simulink model "CM640C_MotAg1Meas"  (R2013b)
settings: Solver=VariableStepDiscrete  SolverMode=SingleTasking  StartTime=0.0  StopTime=1  FixedStep=0.002  RelTol=1e-3
values from neighbouring files (symbols this model uses):
  ARCHGLBPRM_2PI_ULS_F32 = DataDict.Constant    [CM640C_MotAg1Meas_DataDict.m]
  CNTPERREV_MOTREV_S15P16 = DataDict.Constant    [CM640C_MotAg1Meas_DataDict.m]
  COEFFTBLELMSIZE_CNT_U08 = DataDict.Constant    [CM640C_MotAg1Meas_DataDict.m]
  COEFFTBLSIZE_CNT_U08 = DataDict.Constant    [CM640C_MotAg1Meas_DataDict.m]
  CORRNTBLAGSTEPSIZE_MATRAD_F32 = DataDict.Constant    [CM640C_MotAg1Meas_DataDict.m]
  CORRNTBLSIDXOFFS_CNT_U16 = DataDict.Constant    [CM640C_MotAg1Meas_DataDict.m]
  CORRNTBLSIZE_CNT_U16 = DataDict.Constant    [CM640C_MotAg1Meas_DataDict.m]
  CORRNTBLSIZEMASK_CNT_U08 = DataDict.Constant    [CM640C_MotAg1Meas_DataDict.m]
  MOTAG1ERRTHD_MOTREV_U0P16 = DataDict.Constant    [CM640C_MotAg1Meas_DataDict.m]
  MotAg1MeasMotAgOffs = DataDict.Calibration    [CM640C_MotAg1Meas_DataDict.m]
  MotAg1PrtclFlt = DataDict.NTC    [CM640C_MotAg1Meas_DataDict.m]
  MOTAG1PRTCLFLTFAILSTEP_CNT_U16 = DataDict.Constant    [CM640C_MotAg1Meas_DataDict.m]
  MOTAG1PRTCLFLTPASSSTEP_CNT_U16 = DataDict.Constant    [CM640C_MotAg1Meas_DataDict.m]
  MOTAGCPTLIMFLTMASK_CNT_U32 = DataDict.Constant    [CM640C_MotAg1Meas_DataDict.m]
  MOTAGDELTAPERCORRNPT_CNT_U16 = DataDict.Constant    [CM640C_MotAg1Meas_DataDict.m]
  MOTAGFLTMASK_CNT_U32 = DataDict.Constant    [CM640C_MotAg1Meas_DataDict.m]
  MOTAGIDXMASK_CNT_U16 = DataDict.Constant    [CM640C_MotAg1Meas_DataDict.m]
  MOTAGLIMMASK_CNT_S32 = DataDict.Constant    [CM640C_MotAg1Meas_DataDict.m]
  MOTAGMGNLIMFLTMASK_CNT_U32 = DataDict.Constant    [CM640C_MotAg1Meas_DataDict.m]
  MOTAGMINWAITPERD_CNT_U32 = DataDict.Constant    [CM640C_MotAg1Meas_DataDict.m]
  MOTAGOFFS_CNT_S32 = DataDict.Constant    [CM640C_MotAg1Meas_DataDict.m]
  MOTAGOVFFLTMASK_CNT_U32 = DataDict.Constant    [CM640C_MotAg1Meas_DataDict.m]
  MOTAGSPITRSMMASK_CNT_U32 = DataDict.Constant    [CM640C_MotAg1Meas_DataDict.m]
  MOTAGVLTGFLTMASK_CNT_U32 = DataDict.Constant    [CM640C_MotAg1Meas_DataDict.m]
  NOMOTAGFLTMASK_CNT_U32 = DataDict.Constant    [CM640C_MotAg1Meas_DataDict.m]
  READBUFADR_CNT_U32 = DataDict.Constant    [CM640C_MotAg1Meas_DataDict.m]
  READBUFIDX_CNT_U08 = DataDict.Constant    [CM640C_MotAg1Meas_DataDict.m]
  SNSRAGMASK_CNT_U32 = DataDict.Constant    [CM640C_MotAg1Meas_DataDict.m]
  SNSRCNTMASK_CNT_U32 = DataDict.Constant    [CM640C_MotAg1Meas_DataDict.m]
  SPIAGCNTREGIDX_CNT_U08 = DataDict.Constant    [CM640C_MotAg1Meas_DataDict.m]
  SPIAGREGIDX_CNT_U08 = DataDict.Constant    [CM640C_MotAg1Meas_DataDict.m]
  SPISTATREGIDX_CNT_U08 = DataDict.Constant    [CM640C_MotAg1Meas_DataDict.m]
  SPITURNCNTRREGIDX_CNT_U08 = DataDict.Constant    [CM640C_MotAg1Meas_DataDict.m]
  STRTPTRINITVAL_CNT_U32 = DataDict.Constant    [CM640C_MotAg1Meas_DataDict.m]
  STRTPTRPERVAL_CNT_U32 = DataDict.Constant    [CM640C_MotAg1Meas_DataDict.m]
  TURNCNTRHALFOFFS_CNT_S16 = DataDict.Constant    [CM640C_MotAg1Meas_DataDict.m]
  TURNCNTROFFS_CNT_S16 = DataDict.Constant    [CM640C_MotAg1Meas_DataDict.m]
  TURNCNTRREGMASK_CNT_U32 = DataDict.Constant    [CM640C_MotAg1Meas_DataDict.m]
  VLDMOTAGFLTMASK_CNT_U32 = DataDict.Constant    [CM640C_MotAg1Meas_DataDict.m]
undefined symbols (not defined in the file or in its folder): NtcSts1, sigbuilder_block
libraries: simulink x41, FloatToFixd x1, NxtrMax x1
(part 1 of 7)
settings Model: RequirementInfo="{}  %GIDa_ca294f38_ed7c_4fb9_8c54_f4d56271bfc7"  ModifiedHistory=Rev 008: Updated model to Matlab 2013B, added comments to show requirement linkage  PauseTimes=0.026  Creator=nz3zln  LastModifiedBy=tz8cy0
settings SolverCC: AutoInsertRateTranBlk=on  InsertRTBMode=Always
settings DataIOCC: LimitDataPoints=off  SaveFormat=Structure  ReturnWorkspaceOutputs=on
settings OptimizationCC: BlockReduction=off  InlineParams=on  ZeroExternalMemoryAtStartup=off  ZeroInternalMemoryAtStartup=off  OptimizeModelRefInitCode=on  LifeSpan=1
settings DebuggingCC: SignalInfNanChecking=error  SignalRangeChecking=warning  UnderspecifiedInitializationDetection=Simplified  SolverPrmCheckMsg=error  InheritedTsInSrcMsg=error  DiscreteInheritContinuousMsg=error  SingleTaskRateTransMsg=error  TasksWithSamePriorityMsg=error  SigSpecEnsureSampleTimeMsg=error  CheckMatrixSingularityMsg=error  ParameterUnderflowMsg=error  ParameterPrecisionLossMsg=error  ParameterTunabilityLossMsg=error  FixptConstUnderflowMsg=warning  FixptConstOverflowMsg=warning  VectorMatrixConversionMsg=error  SignalLabelMismatchMsg=error  UnconnectedInputMsg=error  UnconnectedOutputMsg=error  UnconnectedLineMsg=error  SFcnCompatibilityMsg=error  UniqueDataStoreMsg=warning  BusObjectLabelMismatch=error  RootOutportRequireBusObject=error  AssertControl=DisableAll  ModelReferenceIOMsg=error  ModelReferenceVersionMismatchMessage=warning  ModelReferenceIOMismatchMessage=error  ModelReferenceCSMismatchMessage=warning  ModelReferenceDataLoggingMessage=error  StateNameClashWarn=warning  StrictBusMsg=ErrorOnBusTreatedAsVector  NonBusSignalsTreatedAsBus=error  SFUnexpectedBacktrackingDiag=error  SFInvalidInputDataAccessInChartInitDiag=error  SFNoUnconditionalDefaultTransitionDiag=error  SFTransitionOutsideNaturalParentDiag=error  SFUnconditionalTransitionShadowingDiag=error  SFUndirectedBroadcastEventsDiag=error
settings ModelReferenceCC: ModelReferenceNumInstancesAllowed=Single
settings RTWCC: SystemTargetFile=autosar.tlc  GenCodeOnly=on  TemplateMakefile=ert_default_tmf  Description=AUTOSAR  GenerateReport=on  ProcessScript=autosar_make_rtw_hook  LaunchReport=on
settings CodeAppCC: GenerateComments=off  IgnoreCustomStorageClasses=off  CustomSymbolStrType=$N$R$M  CustomSymbolStrBlkIO=$N$M  SimulinkBlockComments=off
settings STFCustomTargetCC: ParMdlRefBuildCompliant=on  CompOptLevelCompliant=on  IncludeMdlTerminateFcn=off  CombineOutputUpdateFcns=on  SuppressErrorStatus=on  ERTFirstTimeCompliant=on  ERTCustomFileBanners=on  SupportNonFinite=off  SupportComplex=off  SupportContinuousTime=off  SupportNonInlinedSFcns=off  MATLABClassNameForMDSCustomization=Simulink.SoftwareTarget.ERTCustomization  AutosarCompliant=on  GRTInterface=off  SystemTargetFile=autosar.tlc
settings ERTTargetCC: CodeReplacementLibrary=ANSI_C  ConcurrentExecutionCompliant=off  IncludeMdlTerminateFcn=off  SuppressErrorStatus=on  SupportNonFinite=off  SupportComplex=off  ModelStepFunctionPrototypeControlCompliant=off  CPPClassGenCompliant=off  AutosarCompliant=on  InlinedParameterPlacement=NonHierarchical  ERTCustomFileTemplate=example_file_process.tlc  EnableUserReplacementTypes=on

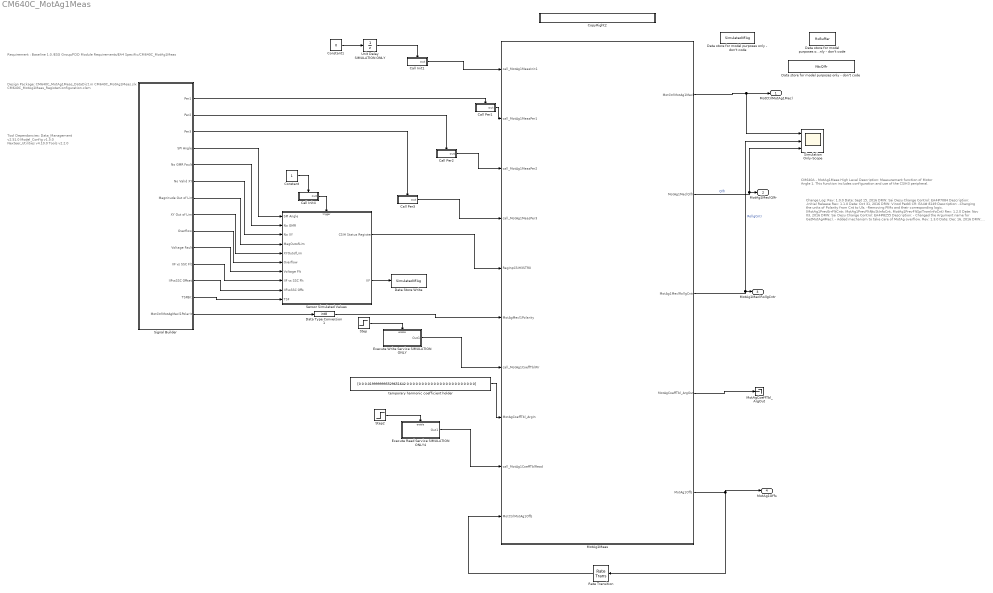
== system CM640C_MotAg1Meas ==
  note: Requirement : Baseline 1.0
      | /ESG Group/FDD Module Requirements/EA4 Specific/CM640C_MotAg1Meas
  note: Tool Dependancies:
      | Data_Management v2.51.0
      | Model_Config v1.5.0
      | Nexteer_Utilities v4.10.0
      | Tools v2.2.0
  note: Design Package:
      | CM640C_MotAg1Meas_DataDict.m
      | CM640C_MotAg1Meas.slx
      | CM640C_MotAg1Meas_RegisterConfiguration.xlsm
  note: Change Log:
      |
      | Rev: 1.0.0
      | Date: Sept 15, 2016
      | DRW: Sai Desu
      | Change Control: EA4#7084
      | Description:
      | -Initial Release
      |
      | Rev: 1.1.0
      | Date: Oct 31, 2016
      | DRW: Vinod Peddi
      | CR: EA4# 8149
      | Description:
      | -Changing the units of Polarity from Cnt to Uls.
      | -Removing PIMs and their corresponding logic. (MotAg1PrevErrFltCntr,
      | MotAg1PrevFltNtcStInfoCnt, MotAg1PrevFltSpiTrsmInfoCnt)
      |
      | Rev: 1.2.0
      | Date: Nov 03, 2016
      | DRW: Sai Desu
      | Change Control: EA4#8255
      | Description:
      | - Changed the Argument name for GetMotAg4Mecl.
      | - Added mechanism to take care of MotAg overflow.
      |
      | Rev: 1.3.0
      | Date: Dec 16, 2016
      | DRW: Peddi
      | CR: EA4# 8965
      | Description:
      | Changes to the Tx buffer.
      | Start pointer of Tx buffer changed (Both Per and Init)
      | Start pointer of the Rx changed.
      | Read the Rx register only once in the for loop. Write the local variable to the Display variable (Per2)
      | Added MotAg1MeasMotAgOffs in Per 2 Diagnostics block. MotAg1MeasMotAgOffs = 0.5
      |
      | Rev: 1.4.0
      | Date: Dec 21, 2016
      | DRW: Erlenbeck
      | CR: EA4# 9018
      | Description:
      | Modified logic to normalize motor angle for an instance that had unreachable code
      |
      | Rev: 1.5.0
      | Date: Jan 18, 2017
      | DRW: Peddi
      | CR: EA4#9380 Anomoly fix EA4#9381
      | Description:
      | ~ Added  a PIM to provide a mechanism to synchronize the data between IIF and SPI angle.
      | ~ Added a display variable to log the delta between IIF and SPI angle
  note: CM640A - MotAg1Meas
      |
      | High Level Description:
      | Measurement function of Motor Angle 1.  This function includes configuration
      | and use of the CSIH3 peripheral.
  Call Init1 : Subsystem  TreatAsAtomicUnit=on
  Call Init4 : Subsystem  TreatAsAtomicUnit=on
  Call Per1 : Subsystem  TreatAsAtomicUnit=on
  Call Per2 : Subsystem  TreatAsAtomicUnit=on
  Call Per3 : Subsystem  TreatAsAtomicUnit=on
  Constant : Constant  OutDataTypeStr=boolean
  Constant1 : Constant  Value=0  OutDataTypeStr=uint8
  CopyRight2 : Subsystem  Description=|  mask(Copyright Information){none=on}
      | Copyright info block.                                               
      |                                                                     
      | Place copyright information at the top of every subsystem in design.
      mask prompts: none "No parameters"
      mask help: Place copyright information at the top of every subsystem in design.
      mask Display:
      | NxtrConf = 'Nexteer Confidential';
      | 
      | sys = bdroot; %handle for the current model ("system")
      | first = get_param(sys,'Created');
      | first = first(end-3:end);  %year is last four digits
      | 
      | last = get_param(sys,'LastModifiedDate');
      | if isempty(last)
      |     last = datestr(now,'yyyy');
      | else
      |     last = last(end-3:end);
      | end
      | 
      | if strcmp(first,last)
      |     fprintf('%s -- Copyright %s Nexteer',NxtrConf,first)
      | else
      |     fprintf('%s -- %s%s- %s Nexteer',NxtrConf,char(169),first,last)
      | end
  Data Store Write : DataStoreWrite  DataStoreName=SimulatedIIFAg
  Data Type Conversion1 : DataTypeConversion  OutDataTypeStr=int8
  Data store for model purposes only - don't code : DataStoreMemory  DataStoreName=NtcQlfr  ReadBeforeWriteMsg=warning  WriteAfterWriteMsg=warning  WriteAfterReadMsg=warning
  "Data store for model purposes only - don't code " : DataStoreMemory  DataStoreName=SimulatedIIFAg
  "Data store for model purposes only - don't code  " : DataStoreMemory  DataStoreName=RxBuffer  InitialValue=zeros(1,10)
  Execute Read Service SIMULATION ONLY4 : Subsystem  TreatAsAtomicUnit=on
  Execute Write Service SIMULATION ONLY : Subsystem  TreatAsAtomicUnit=on
  MotAg1Meas : Subsystem
  MotAgCoeffTbl_ArgOut : Terminator
  Rate Transition : RateTransition
  Sensor Simulated Values : Subsystem
  Signal Builder : Subsystem  Tag=STV Subsys  LoadFcn=sigbuilder_block('load');  StartFcn=sigbuilder_block('start');  StopFcn=sigbuilder_block('stop');  ClipboardFcn=sigbuilder_block('clipboard');  mask(Sigbuilder block){}
      mask help: Simulink:masks:SigbuilderBlock_MD
      mask init:
      | if ~strcmp(get_param(bdroot(gcbh),'SimulationStatus'),'stopped') tuvar = sigbuilder_block('maskInit'); end
      settings: CopyFcn=sigbuilder_block('copy');  DeleteFcn=sigbuilder_block('delete');  ModelCloseFcn=sigbuilder_block('modelClose');  PreSaveFcn=sigbuilder_block('preSave');  PauseFcn=sigbuilder_block('pause');  ContinueFcn=sigbuilder_block('continue');  NameChangeFcn=sigbuilder_block('namechange');  OpenFcn=sigbuilder_block('open',[0 31.6552 1024.14 488.483 ]);  CloseFcn=sigbuilder_block('close');
      mask Display: plot(0, 0, 100, 100,[2, 2, 32, 32, 2], [68, 8, 8, 68, 68],[32, 2], [38, 38], [32, 19, 2],[53, 60, 44], [32, 17, 17, 2],[16, 16, 31, 31]);txt = getActiveGroup(gcbh);text(2, 100, txt,'verticalAlignment', 'top');
  Simulation Only-Scope : Scope  NumInputPorts=3
      settings: YMin=-5~-5~-5  YMax=5~5~5  SaveName=ScopeData4
  Step : Step  Time=0.05  SampleTime=0
  Step2 : Step  Time=0.8  SampleTime=0
  Unit Delay SIMULATION ONLY : UnitDelay  InitialCondition=1  SampleTime=-1
  temporary harmonic coefficient holder : Constant  Value=[0 0 0.0199999995529651642 0 0 0 0 0 0 0 0 0 0 0 0 0 0 0 0 0 0 0 0 0 0 0]  OutDataTypeStr=single
  MotCtrlMotAg1Mecl : Outport
  MotAg1MeclQlfr : Outport  RequirementInfo={} %GIDa_67900831_6cb3_4e4b_960b_3d75fb5cf41f  Port=2
  MotAg1MeclRollgCntr : Outport  RequirementInfo={} %GIDa_42bff207_af2f_4bdf_9154_81e061bb0eb3  Port=3
  MotAg1Offs : Outport  Port=4
  wires:
  Call Init1/1(out) -> MotAg1Meas/1(call_MotAg1MeasInit1)
  Call Per1/1(out) -> MotAg1Meas/2(call_MotAg1MeasPer1)
  Call Init4/1(out) -> Sensor Simulated Values/Trigger
  Call Per2/1(out) -> MotAg1Meas/3(call_MotAg1MeasPer2)
  Signal Builder/4(SPI Angle) -> Sensor Simulated Values/1(SPI Angle)
  Signal Builder/5(No GMR Fault) -> Sensor Simulated Values/2(No GMR)
  Signal Builder/6(No Valid XY) -> Sensor Simulated Values/3(No XY)
  Signal Builder/7(Magnitude Out of Lim) -> Sensor Simulated Values/4(MagOutofLim)
  Signal Builder/8(XY Out of Lim) -> Sensor Simulated Values/5(XYOutofLim)
  Signal Builder/9(Overflow) -> Sensor Simulated Values/6(Overflow)
  Signal Builder/10(Voltage Fault) -> Sensor Simulated Values/7(Voltage Flt)
  Signal Builder/14(MotCtrlMotAgMecl1Polarity) -> Data Type Conversion1/1
  Signal Builder/11(IIF vs SSC Flt) -> Sensor Simulated Values/8(IIF vs SSC Flt)
  MotAg1Meas/1(MotCtrlMotAg1Mecl) -> Simulation Only-Scope/1, MotCtrlMotAg1Mecl/1
  MotAg1Meas/2(MotAg1MeclQlfr) -> Simulation Only-Scope/3, MotAg1MeclQlfr/1  "Qlfr"
  MotAg1Meas/3(MotAg1MeclRollgCntr) -> Simulation Only-Scope/2, MotAg1MeclRollgCntr/1  "RollgCntr"
  Call Per3/1(out) -> MotAg1Meas/4(call_MotAg1MeasPer3)
  Sensor Simulated Values/2(IIF) -> Data Store Write/1
  Signal Builder/1(Per1) -> Call Per1/Enable
  Signal Builder/2(Per2) -> Call Per2/Enable
  Signal Builder/3(Per3) -> Call Per3/Enable
  Constant/1 -> Call Init4/Enable
  Step/1 -> Execute Write Service SIMULATION ONLY/Enable
  Execute Write Service SIMULATION ONLY/1(Out1) -> MotAg1Meas/7(call_MotAg1CoeffTblWr)
  Step2/1 -> Execute Read Service SIMULATION ONLY4/Enable
  Execute Read Service SIMULATION ONLY4/1(Out1) -> MotAg1Meas/9(call_MotAg1CoeffTblRead)
  temporary harmonic coefficient holder/1 -> MotAg1Meas/8(MotAgCoeffTbl_ArgIn)
  Data Type Conversion1/1 -> MotAg1Meas/6(MotAgMecl1Polarity)
  MotAg1Meas/4(MotAgCoeffTbl_ArgOut) -> MotAgCoeffTbl_ArgOut/1
  Constant1/1 -> Unit Delay SIMULATION ONLY/1
  Unit Delay SIMULATION ONLY/1 -> Call Init1/Enable
  Sensor Simulated Values/1(CSIH Status Register) -> MotAg1Meas/5(RegInpCSIH3STR0)
  Signal Builder/12(IIFvsSSC Offset) -> Sensor Simulated Values/9(IIFvsSSC Offs)
  MotAg1Meas/5(MotAg1Offs) -> MotAg1Offs/1, Rate Transition/1
  Rate Transition/1 -> MotAg1Meas/10(MotCtrlMotAg1Offs)
  Signal Builder/13(TSFBit) -> Sensor Simulated Values/10(TSF)

== system CM640C_MotAg1Meas/Call Init1 ==
  Enable : EnablePort
  Function Call Trigger : simulink/Ports & Subsystems/Function-Call Generator  RequirementInfo={} %GIDa_a6a4a62e_0f67_4a31_8bd8_36e712ec7718  sample_time=0.002  numberOfIterations=1
  out : Outport
  wires:
  Function Call Trigger/1 -> out/1

== system CM640C_MotAg1Meas/Call Init4 ==
  Enable : EnablePort
  Function Call Trigger : simulink/Ports & Subsystems/Function-Call Generator  RequirementInfo={} %GIDa_e4718f48_eca1_4e3b_a34c_2e87126956e6  sample_time=0.0005  numberOfIterations=1
  out : Outport
  wires:
  Function Call Trigger/1 -> out/1

== system CM640C_MotAg1Meas/Call Per1 ==
  Enable : EnablePort
  Function Call Trigger : simulink/Ports & Subsystems/Function-Call Generator  RequirementInfo={} %GIDa_24fcf975_4917_4f1f_849b_092f4c8c017b  sample_time=0.0005  numberOfIterations=1
  out : Outport
  wires:
  Function Call Trigger/1 -> out/1

== system CM640C_MotAg1Meas/Call Per2 ==
  Enable : EnablePort
  Function Call Trigger : simulink/Ports & Subsystems/Function-Call Generator  RequirementInfo={} %GIDa_282a9b6d_d37e_41e8_9e51_956de398018d  sample_time=0.002  numberOfIterations=1
  out : Outport
  wires:
  Function Call Trigger/1 -> out/1

== system CM640C_MotAg1Meas/Call Per3 ==
  Enable : EnablePort
  Function Call Trigger : simulink/Ports & Subsystems/Function-Call Generator  RequirementInfo={} %GIDa_e014509a_348b_4b3c_b206_d74a871c47c1  sample_time=0.002  numberOfIterations=1
  out : Outport
  wires:
  Function Call Trigger/1 -> out/1

== system CM640C_MotAg1Meas/CopyRight2 ==

== system CM640C_MotAg1Meas/Execute Read Service SIMULATION ONLY4 ==
  Enable : EnablePort
  Function-Call Generator1 : simulink/Ports & Subsystems/Function-Call Generator  sample_time=0.0000625  numberOfIterations=1
  Out1 : Outport
  wires:
  Function-Call Generator1/1 -> Out1/1

== system CM640C_MotAg1Meas/Execute Write Service SIMULATION ONLY ==
  Enable : EnablePort
  Function-Call Generator1 : simulink/Ports & Subsystems/Function-Call Generator  sample_time=0.0000625  numberOfIterations=1
  Out1 : Outport
  wires:
  Function-Call Generator1/1 -> Out1/1

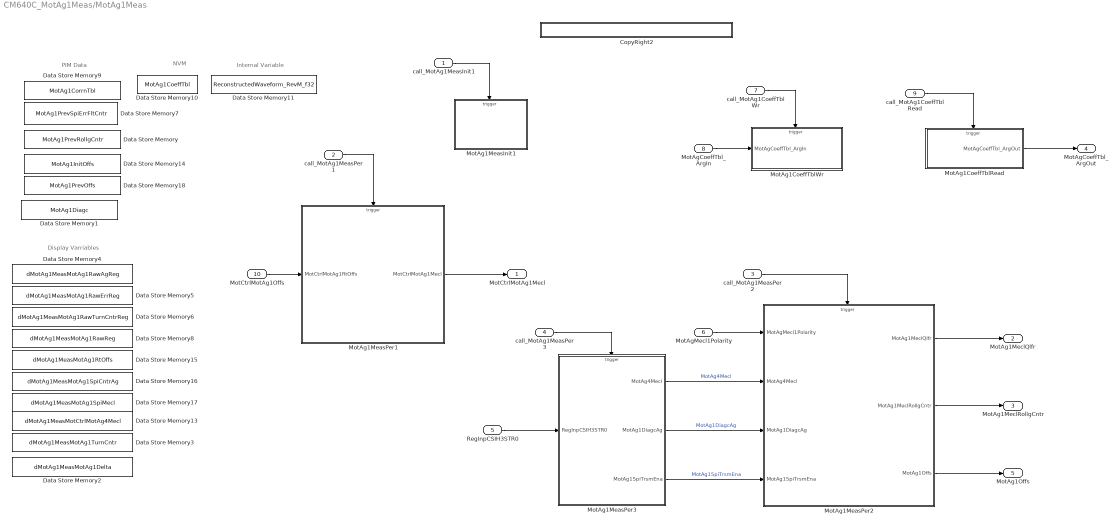
== system CM640C_MotAg1Meas/MotAg1Meas ==
  note: Internal Variable
  note: NVM
  note: Display Varriables
  note: PIM Data
  call_MotAg1MeasInit1 : Inport  RequirementInfo={} %GIDa_aa3d25db_0abc_4b4b_8e52_ac4f5fb50d13
  call_MotAg1MeasPer1 : Inport  RequirementInfo={} %GIDa_24a857ea_f67c_41e3_b28e_796ae3f2df8f  Port=2
  call_MotAg1MeasPer2 : Inport  RequirementInfo={} %GIDa_114ad00e_fb09_47ae_915a_70bc97bf101b  Port=3
  call_MotAg1MeasPer3 : Inport  RequirementInfo={} %GIDa_6882562e_ed69_4bbf_a902_64b38fcece32  Port=4
  RegInpCSIH3STR0 : Inport  Port=5
  MotAgMecl1Polarity : Inport  Port=6
  call_MotAg1CoeffTblWr : Inport  RequirementInfo={} %GIDa_a4ef14fd_eb48_479c_b906_507c8cb8087a  Port=7
  MotAgCoeffTbl_ArgIn : Inport  RequirementInfo={} %GIDa_da95f0f4_69a7_46bf_ae04_bb2228fda533  Port=8
  call_MotAg1CoeffTblRead : Inport  RequirementInfo={} %GIDa_4d6d5774_6a08_451d_8083_e45c8119ea4c  Port=9
  MotCtrlMotAg1Offs : Inport  RequirementInfo={} %GIDa_ad82f0fa_baae_4b47_8664_e0c35af22a8f  Port=10
  CopyRight2 : Subsystem  Description=|  mask(Copyright Information){none=on}
      | Copyright info block.                                               
      |                                                                     
      | Place copyright information at the top of every subsystem in design.
      mask prompts: none "No parameters"
      mask help: Place copyright information at the top of every subsystem in design.
      mask Display:
      | NxtrConf = 'Nexteer Confidential';
      | 
      | sys = bdroot; %handle for the current model ("system")
      | first = get_param(sys,'Created');
      | first = first(end-3:end);  %year is last four digits
      | 
      | last = get_param(sys,'LastModifiedDate');
      | if isempty(last)
      |     last = datestr(now,'yyyy');
      | else
      |     last = last(end-3:end);
      | end
      | 
      | if strcmp(first,last)
      |     fprintf('%s -- Copyright %s Nexteer',NxtrConf,first)
      | else
      |     fprintf('%s -- %s%s- %s Nexteer',NxtrConf,char(169),first,last)
      | end
  Data Store Memory : DataStoreMemory  DataStoreName=MotAg1PrevRollgCntr  StateMustResolveToSignalObject=on
  Data Store Memory1 : DataStoreMemory  DataStoreName=MotAg1Diagc  StateMustResolveToSignalObject=on
  Data Store Memory10 : DataStoreMemory  DataStoreName=MotAg1CoeffTbl  InitialValue=[]  StateMustResolveToSignalObject=on
  Data Store Memory11 : DataStoreMemory  DataStoreName=ReconstructedWaveform_RevM_f32  InitialValue=zeros(128,1)  OutDataTypeStr=single
  Data Store Memory13 : DataStoreMemory  RequirementInfo={} %GIDa_4e82f34d_86fb_4935_bcb8_034c8e3546d0  DataStoreName=dMotAg1MeasMotCtrlMotAg4Mecl  StateMustResolveToSignalObject=on
  Data Store Memory14 : DataStoreMemory  DataStoreName=MotAg1InitOffs  StateMustResolveToSignalObject=on
  Data Store Memory15 : DataStoreMemory  RequirementInfo={} %GIDa_2b1b264b_8711_4ba6_8f68_2cd4c37da107  DataStoreName=dMotAg1MeasMotAg1RtOffs  StateMustResolveToSignalObject=on
  Data Store Memory16 : DataStoreMemory  RequirementInfo={} %GIDa_aec4d6d4_6033_4799_883f_72c67c7c18a3  DataStoreName=dMotAg1MeasMotAg1SpiCntrAg  StateMustResolveToSignalObject=on
  Data Store Memory17 : DataStoreMemory  RequirementInfo={} %GIDa_6f348a9f_6a23_4e53_a6dc_a9321998a2b3  DataStoreName=dMotAg1MeasMotAg1SpiMecl  StateMustResolveToSignalObject=on
  Data Store Memory18 : DataStoreMemory  DataStoreName=MotAg1PrevOffs  StateMustResolveToSignalObject=on
  Data Store Memory2 : DataStoreMemory  RequirementInfo={} %GIDa_02071296_bcba_4272_947f_9380dbb96bc9  DataStoreName=dMotAg1MeasMotAg1Delta  StateMustResolveToSignalObject=on
  Data Store Memory3 : DataStoreMemory  RequirementInfo={} %GIDa_95d3f51e_919f_43c4_a708_f9e2d558fa00  DataStoreName=dMotAg1MeasMotAg1TurnCntr  StateMustResolveToSignalObject=on
  Data Store Memory4 : DataStoreMemory  RequirementInfo={} %GIDa_e62aa2d5_70fa_4cdf_9fa5_a8ab759b7de5  DataStoreName=dMotAg1MeasMotAg1RawAgReg  StateMustResolveToSignalObject=on
  Data Store Memory5 : DataStoreMemory  RequirementInfo={} %GIDa_9a41dc83_29ae_4514_8647_225ad4cf8550  DataStoreName=dMotAg1MeasMotAg1RawErrReg  StateMustResolveToSignalObject=on
  Data Store Memory6 : DataStoreMemory  RequirementInfo={} %GIDa_c9ec4852_d1ef_4f73_8864_5550a24c73a6  DataStoreName=dMotAg1MeasMotAg1RawTurnCntrReg  StateMustResolveToSignalObject=on
  Data Store Memory7 : DataStoreMemory  DataStoreName=MotAg1PrevSpiErrFltCntr  StateMustResolveToSignalObject=on
  Data Store Memory8 : DataStoreMemory  RequirementInfo={} %GIDa_5539a78e_8c30_4b51_8353_f520af13ac20  DataStoreName=dMotAg1MeasMotAg1RawReg  InitialValue=[]  StateMustResolveToSignalObject=on
  Data Store Memory9 : DataStoreMemory  DataStoreName=MotAg1CorrnTbl  InitialValue=[]  StateMustResolveToSignalObject=on
  MotAg1CoeffTblRead : Subsystem  RequirementInfo="{'linktype_rmi_doors' '00011b54 (/ESG Group/FDD Module Requirements/EA4 Specific/CM640C_MotAg1Meas)' '#CM640C_81' 'true' 'REQ:  CM640C_81' '' } %GIDa_7461cfd5_d880_40a9_a2ef_3584dfe541c9"
  MotAg1CoeffTblWr : Subsystem  RequirementInfo="{'linktype_rmi_doors' '00011b54 (/ESG Group/FDD Module Requirements/EA4 Specific/CM640C_MotAg1Meas)' '#CM640C_32' 'true' 'REQ:  CM640C_32' '' } %GIDa_bc26aedd_e004_48b3_8c67_ec36ea15062c"
  MotAg1MeasInit1 : Subsystem  RequirementInfo={} %GIDa_23158868_3489_495a_8114_4f4d0466d444
  MotAg1MeasPer1 : Subsystem  TreatAsAtomicUnit=on
  MotAg1MeasPer2 : Subsystem  TreatAsAtomicUnit=on
  MotAg1MeasPer3 : Subsystem
  MotCtrlMotAg1Mecl : Outport
  MotAg1MeclQlfr : Outport  RequirementInfo={} %GIDa_17ff9147_53fc_4340_8d34_b5d142602724  Port=2
  MotAg1MeclRollgCntr : Outport  RequirementInfo={} %GIDa_b32774aa_4d8d_4c20_84bb_a6144a3fdec3  Port=3
  MotAgCoeffTbl_ArgOut : Outport  Port=4
  MotAg1Offs : Outport  Port=5
  wires:
  call_MotAg1MeasInit1/1 -> MotAg1MeasInit1/Trigger
  call_MotAg1MeasPer2/1 -> MotAg1MeasPer2/Trigger
  call_MotAg1MeasPer1/1 -> MotAg1MeasPer1/Trigger
  MotAg1MeasPer1/1(MotCtrlMotAg1Mecl) -> MotCtrlMotAg1Mecl/1
  MotAgMecl1Polarity/1 -> MotAg1MeasPer2/1(MotAgMecl1Polarity)
  MotAg1MeasPer2/1(MotAg1MeclQlfr) -> MotAg1MeclQlfr/1
  MotAg1MeasPer2/2(MotAg1MeclRollgCntr) -> MotAg1MeclRollgCntr/1
  call_MotAg1MeasPer3/1 -> MotAg1MeasPer3/Trigger
  call_MotAg1CoeffTblWr/1 -> MotAg1CoeffTblWr/Trigger
  MotAgCoeffTbl_ArgIn/1 -> MotAg1CoeffTblWr/1(MotAgCoeffTbl_ArgIn)
  call_MotAg1CoeffTblRead/1 -> MotAg1CoeffTblRead/Trigger
  MotAg1CoeffTblRead/1(MotAgCoeffTbl_ArgOut) -> MotAgCoeffTbl_ArgOut/1
  RegInpCSIH3STR0/1 -> MotAg1MeasPer3/1(RegInpCSIH3STR0)
  MotAg1MeasPer2/3(MotAg1Offs) -> MotAg1Offs/1
  MotCtrlMotAg1Offs/1 -> MotAg1MeasPer1/1(MotCtrlMotAg1RtOffs)
  MotAg1MeasPer3/1(MotAg4Mecl) -> MotAg1MeasPer2/2(MotAg4Mecl)  "MotAg4Mecl"
  MotAg1MeasPer3/3(MotAg1SpiTrsmEna) -> MotAg1MeasPer2/4(MotAg1SpiTrsmEna)  "MotAg1SpiTrsmEna"
  MotAg1MeasPer3/2(MotAg1DiagcAg) -> MotAg1MeasPer2/3(MotAg1DiagcAg)  "MotAg1DiagcAg"

== system CM640C_MotAg1Meas/Sensor Simulated Values ==
  note: 0 = ReadSTAT
      | 1 = CSQDeselect
      | 2 = WriteCmd12
      | 3 = ReadAVAL
      | 4 = CSQDeselect
      | 5 = WriteCmd13
      | 6 = ReadAREV
      | 7 = CSQDeselect
      | 8 = WriteCmd14
      | 9 = ReadIIFCNT
  SPI Angle : Inport
  No GMR : Inport  Port=2
  No XY : Inport  Port=3
  MagOutofLim : Inport  Port=4
  XYOutofLim : Inport  Port=5
  Overflow : Inport  Port=6
  Voltage Flt : Inport  Port=7
  IIF vs SSC Flt : Inport  Port=8
  IIFvsSSC Offs : Inport  Port=9
  TSF : Inport  Port=10
  function : TriggerPort  TriggerType=function-call
  Constant : Constant  Value=0
  CopyRight2 : Subsystem  Description=|  mask(Copyright Information){none=on}
      | Copyright info block.                                               
      |                                                                     
      | Place copyright information at the top of every subsystem in design.
      mask prompts: none "No parameters"
      mask help: Place copyright information at the top of every subsystem in design.
      mask Display:
      | NxtrConf = 'Nexteer Confidential';
      | 
      | sys = bdroot; %handle for the current model ("system")
      | first = get_param(sys,'Created');
      | first = first(end-3:end);  %year is last four digits
      | 
      | last = get_param(sys,'LastModifiedDate');
      | if isempty(last)
      |     last = datestr(now,'yyyy');
      | else
      |     last = last(end-3:end);
      | end
      | 
      | if strcmp(first,last)
      |     fprintf('%s -- Copyright %s Nexteer',NxtrConf,first)
      | else
      |     fprintf('%s -- %s%s- %s Nexteer',NxtrConf,char(169),first,last)
      | end
  Data Store Write : DataStoreWrite  DataStoreName=RxBuffer
  Data Type Conversion : DataTypeConversion  OutDataTypeStr=uint32
  Mux : Mux  Inputs=10
  Signal Processing : Subsystem
  CSIH Status Register : Outport
  IIF : Outport  Port=2
  wires:
  SPI Angle/1 -> Signal Processing/1(Angle value)
  No GMR/1 -> Signal Processing/2(No GMR)
  No XY/1 -> Signal Processing/3(No XY)
  MagOutofLim/1 -> Signal Processing/4(MagOutofLim)
  XYOutofLim/1 -> Signal Processing/5(XYOutofLim)
  Overflow/1 -> Signal Processing/6(Overflow)
  Voltage Flt/1 -> Signal Processing/7(Voltage Flt)
  IIF vs SSC Flt/1 -> Signal Processing/8(IIF vs SSC Flt)
  IIFvsSSC Offs/1 -> Signal Processing/9(IIFvsSSC Offs)
  Signal Processing/5(EncaAngle) -> IIF/1
  Signal Processing/6(RegOut) -> CSIH Status Register/1
  Constant/1 -> Mux/9, Mux/8, Mux/6, Mux/5, Mux/3, Mux/2
  Mux/1 -> Data Type Conversion/1
  Data Type Conversion/1 -> Data Store Write/1
  TSF/1 -> Signal Processing/10(TSF)
  Signal Processing/1(StatReg) -> Mux/1
  Signal Processing/2(AgReg) -> Mux/4
  Signal Processing/3(TurnCntr) -> Mux/7
  Signal Processing/4(SpiCnt) -> Mux/10

== system CM640C_MotAg1Meas/Signal Builder ==
  Demux : Demux  Tag=STV Demux  Outputs=14
  FromWs : FromWorkspace  Tag=STV FromWs  VariableName=tuvar  SampleTime=0
      SigBuilderData=|
      | common.afterFinalStr = 'Extrapolate'
      | common.sampleTime = 0
      | dataSet(1).timeRange = [0 1]
      | dataSet(1).name = 'No Fault'
      | dataSet(2).timeRange = [0 1]
      | dataSet(2).name = 'Fault'
      | dataSet(3).timeRange = [0 1]
      | dataSet(3).name = 'ExtendedFlt'
      | dataSet(4).timeRange = [0 1]
      | dataSet(4).name = 'Polarity Check'
      | dataSet(5).timeRange = [0 1]
      | dataSet(5).name = 'Fault1'
      | dataSet(6).timeRange = [0 1]
      | dataSet(6).name = 'Offset Compensation'
      | sbobj.Groups(1).Name = 'No Fault'
      | sbobj.Groups(1).Signals(1).Name = 'Per1'
      | sbobj.Groups(1).Signals(1).XData = [0 1]
      | sbobj.Groups(1).Signals(1).YData = [1 1]
      | sbobj.Groups(1).Signals(2).Name = 'Per2'
      | sbobj.Groups(1).Signals(2).XData = [0 1]
      | sbobj.Groups(1).Signals(2).YData = [1 1]
      | sbobj.Groups(1).Signals(3).Name = 'Per3'
      | sbobj.Groups(1).Signals(3).XData = [0 1]
      | sbobj.Groups(1).Signals(3).YData = [1 1]
      | sbobj.Groups(1).Signals(4).Name = 'SPI Angle'
      | sbobj.Groups(1).Signals(4).XData = [0 0.5 1]
      | sbobj.Groups(1).Signals(4).YData = [0 1410 0]
      | sbobj.Groups(1).Signals(5).Name = 'No GMR Fault'
      | sbobj.Groups(1).Signals(5).XData = [0 0.646 0.991 1]
      | sbobj.Groups(1).Signals(5).YData = [0 0 0 0]
      | sbobj.Groups(1).Signals(6).Name = 'No Valid XY'
      | sbobj.Groups(1).Signals(6).XData = [0 0.677 0.991 1]
      | sbobj.Groups(1).Signals(6).YData = [0 0 0 0]
      | sbobj.Groups(1).Signals(7).Name = 'Magnitude Out of Lim'
      | sbobj.Groups(1).Signals(7).XData = [0 0.724 0.991 1]
      | sbobj.Groups(1).Signals(7).YData = [0 0 0 0]
      | sbobj.Groups(1).Signals(8).Name = 'XY Out of Lim'
      | sbobj.Groups(1).Signals(8).XData = [0 0.777 0.992 1]
      | sbobj.Groups(1).Signals(8).YData = [0 0 0 0]
      | sbobj.Groups(1).Signals(9).Name = 'Overflow'
      | sbobj.Groups(1).Signals(9).XData = [0 0.831 0.992 1]
      | sbobj.Groups(1).Signals(9).YData = [0 0 0 0]
      | sbobj.Groups(1).Signals(10).Name = 'Voltage Fault'
      | sbobj.Groups(1).Signals(10).XData = [0 0.883 0.992 1]
      | sbobj.Groups(1).Signals(10).YData = [0 0 0 0]
      | sbobj.Groups(1).Signals(11).Name = 'IIF vs SSC Flt'
      | sbobj.Groups(1).Signals(11).XData = [0 0.4 0.6 1]
      | sbobj.Groups(1).Signals(11).YData = [0 0 0 0]
      | sbobj.Groups(1).Signals(12).Name = 'IIFvsSSC Offset'
      | sbobj.Groups(1).Signals(12).XData = [0 1]
      | sbobj.Groups(1).Signals(12).YData = [32767 32767]
      | sbobj.Groups(1).Signals(13).Name = 'TSFBit'
      | sbobj.Groups(1).Signals(13).XData = [0 0.4 0.6 1]
      | sbobj.Groups(1).Signals(13).YData = [0 0 0 0]
      | sbobj.Groups(1).Signals(14).Name = 'MotCtrlMotAgMecl0Polarity'
      | sbobj.Groups(1).Signals(14).XData = [0 1]
      | sbobj.Groups(1).Signals(14).YData = [1 1]
      | sbobj.Groups(1).TimeRange = [0 1]
      | sbobj.Groups(2).Name = 'Fault'
      | sbobj.Groups(2).Signals(1).Name = 'Per1'
      | sbobj.Groups(2).Signals(1).XData = [0 0.02 0.02 0.028 1]
      | sbobj.Groups(2).Signals(1).YData = [0 0 1 1 1]
      | sbobj.Groups(2).Signals(2).Name = 'Per2'
      | sbobj.Groups(2).Signals(2).XData = [0 0.026 0.026 0.028 1]
      | sbobj.Groups(2).Signals(2).YData = [0 0 1 1 1]
      | sbobj.Groups(2).Signals(3).Name = 'Per3'
      | sbobj.Groups(2).Signals(3).XData = [0 0.026 0.026 0.05 1]
      | sbobj.Groups(2).Signals(3).YData = [0 0 1 1 1]
      | sbobj.Groups(2).Signals(4).Name = 'SPI Angle'
      | sbobj.Groups(2).Signals(4).XData = [0 1]
      | sbobj.Groups(2).Signals(4).YData = [0 1000]
      | sbobj.Groups(2).Signals(5).Name = 'No GMR Fault'
      | sbobj.Groups(2).Signals(5).XData = [0 0.122 0.122 0.477 0.477 1]
      | sbobj.Groups(2).Signals(5).YData = [0 0 1 1 0 0]
      | sbobj.Groups(2).Signals(6).Name = 'No Valid XY'
      | sbobj.Groups(2).Signals(6).XData = [0 0.259 0.259 0.272 0.272 1]
      | sbobj.Groups(2).Signals(6).YData = [0 0 1 1 0 0]
      | sbobj.Groups(2).Signals(7).Name = 'Magnitude Out of Lim'
      | sbobj.Groups(2).Signals(7).XData = [0 0.335 0.335 0.345 0.345 1]
      | sbobj.Groups(2).Signals(7).YData = [0 0 1 1 0 0]
      | sbobj.Groups(2).Signals(8).Name = 'XY Out of Lim'
      | sbobj.Groups(2).Signals(8).XData = [0 0.381 0.381 0.4 0.4 1]
      | sbobj.Groups(2).Signals(8).YData = [0 0 1 1 0 0]
      | sbobj.Groups(2).Signals(9).Name = 'Overflow'
      | sbobj.Groups(2).Signals(9).XData = [0 0.43 0.43 0.444 0.444 1]
      | sbobj.Groups(2).Signals(9).YData = [0 0 1 1 0 0]
      | sbobj.Groups(2).Signals(10).Name = 'Voltage Fault'
      | sbobj.Groups(2).Signals(10).XData = [0 0.473 0.473 0.49 0.49 1]
      | sbobj.Groups(2).Signals(10).YData = [0 0 1 1 0 0]
      | sbobj.Groups(2).Signals(11).Name = 'IIF vs SSC Flt'
      | sbobj.Groups(2).Signals(11).XData = [0 0.527 0.654 1]
      | sbobj.Groups(2).Signals(11).YData = [0 0 0 0]
      | sbobj.Groups(2).Signals(12).Name = 'IIFvsSSC Offset'
      | sbobj.Groups(2).Signals(12).XData = [0 1]
      | sbobj.Groups(2).Signals(12).YData = [58658.3 58658.3]
      | sbobj.Groups(2).Signals(13).Name = 'TSFBit'
      | sbobj.Groups(2).Signals(13).XData = [0 0.585 0.585 0.649 0.649 1]
      | sbobj.Groups(2).Signals(13).YData = [0 0 128 128 0 0]
      | sbobj.Groups(2).Signals(14).Name = 'MotCtrlMotAgMecl0Polarity'
      | sbobj.Groups(2).Signals(14).XData = [0 0.318 0.528 1]
      | sbobj.Groups(2).Signals(14).YData = [1 1 1 1]
      | sbobj.Groups(2).TimeRange = [0 1]
      | sbobj.Groups(3).Name = 'ExtendedFlt'
      | sbobj.Groups(3).Signals(1).Name = 'Per1'
      | sbobj.Groups(3).Signals(1).XData = [0 0.02 0.02 0.028 1]
      | sbobj.Groups(3).Signals(1).YData = [0 0 1 1 1]
      | sbobj.Groups(3).Signals(2).Name = 'Per2'
      | sbobj.Groups(3).Signals(2).XData = [0 0.021 0.021 0.028 1]
      | sbobj.Groups(3).Signals(2).YData = [0 0 1 1 1]
      | sbobj.Groups(3).Signals(3).Name = 'Per3'
      | sbobj.Groups(3).Signals(3).XData = [0 0.043 0.043 0.05 1]
      | sbobj.Groups(3).Signals(3).YData = [0 0 1 1 1]
      | sbobj.Groups(3).Signals(4).Name = 'SPI Angle'
      | sbobj.Groups(3).Signals(4).XData = [0 1]
      | sbobj.Groups(3).Signals(4).YData = [0 1000]
      | sbobj.Groups(3).Signals(5).Name = 'No GMR Fault'
      | sbobj.Groups(3).Signals(5).XData = [0 0.122 0.122 0.261 0.261 1]
      | sbobj.Groups(3).Signals(5).YData = [0 0 1 1 0 0]
      | sbobj.Groups(3).Signals(6).Name = 'No Valid XY'
      | sbobj.Groups(3).Signals(6).XData = [0 0.259 0.259 0.375 0.375 1]
      | sbobj.Groups(3).Signals(6).YData = [0 0 1 1 0 0]
      | sbobj.Groups(3).Signals(7).Name = 'Magnitude Out of Lim'
      | sbobj.Groups(3).Signals(7).XData = [0 0.335 0.335 0.42 0.42 1]
      | sbobj.Groups(3).Signals(7).YData = [0 0 1 1 0 0]
      | sbobj.Groups(3).Signals(8).Name = 'XY Out of Lim'
      | sbobj.Groups(3).Signals(8).XData = [0 0.381 0.381 0.493 0.493 1]
      | sbobj.Groups(3).Signals(8).YData = [0 0 1 1 0 0]
      | sbobj.Groups(3).Signals(9).Name = 'Overflow'
      | sbobj.Groups(3).Signals(9).XData = [0 0.43 0.43 0.575 0.575 1]
      | sbobj.Groups(3).Signals(9).YData = [0 0 1 1 0 0]
      | sbobj.Groups(3).Signals(10).Name = 'Voltage Fault'
      | sbobj.Groups(3).Signals(10).XData = [0 0.473 0.473 0.617 0.617 1]
      | sbobj.Groups(3).Signals(10).YData = [0 0 1 1 0 0]
      | sbobj.Groups(3).Signals(11).Name = 'IIF vs SSC Flt'
      | sbobj.Groups(3).Signals(11).XData = [0 0.283 0.283 0.327 0.327 1]
      | sbobj.Groups(3).Signals(11).YData = [0 0 1 1 0 0]
      | sbobj.Groups(3).Signals(12).Name = 'IIFvsSSC Offset'
      | sbobj.Groups(3).Signals(12).XData = [0 1]
      | sbobj.Groups(3).Signals(12).YData = [0 0]
      | sbobj.Groups(3).Signals(13).Name = 'TSFBit'
      | sbobj.Groups(3).Signals(13).XData = [0 0.4 0.6 1]
      | sbobj.Groups(3).Signals(13).YData = [0 0 0 0]
      | sbobj.Groups(3).Signals(14).Name = 'MotCtrlMotAgMecl0Polarity'
      | sbobj.Groups(3).Signals(14).XData = [0 0.318 0.528 1]
      | sbobj.Groups(3).Signals(14).YData = [1 1 1 1]
      | sbobj.Groups(3).TimeRange = [0 1]
      | sbobj.Groups(4).Name = 'Polarity Check'
      | sbobj.Groups(4).Signals(1).Name = 'Per1'
      | sbobj.Groups(4).Signals(1).XData = [0 0.004 0.004 1]
      | sbobj.Groups(4).Signals(1).YData = [0 0 1 1]
      | sbobj.Groups(4).Signals(2).Name = 'Per2'
      | sbobj.Groups(4).Signals(2).XData = [0 0.016 0.016 1]
      | sbobj.Groups(4).Signals(2).YData = [0 0 1 1]
      | sbobj.Groups(4).Signals(3).Name = 'Per3'
      | sbobj.Groups(4).Signals(3).XData = [0 0.032 0.032 1]
      | sbobj.Groups(4).Signals(3).YData = [0 0 1 1]
      | sbobj.Groups(4).Signals(4).Name = 'SPI Angle'
      | sbobj.Groups(4).Signals(4).XData = [0 1]
      | sbobj.Groups(4).Signals(4).YData = [0 1000]
      | sbobj.Groups(4).Signals(5).Name = 'No GMR Fault'
      | sbobj.Groups(4).Signals(5).XData = [0 0.646 0.991 1]
      | sbobj.Groups(4).Signals(5).YData = [0 0 0 0]
      | sbobj.Groups(4).Signals(6).Name = 'No Valid XY'
      | sbobj.Groups(4).Signals(6).XData = [0 0.677 0.991 1]
      | sbobj.Groups(4).Signals(6).YData = [0 0 0 0]
      | sbobj.Groups(4).Signals(7).Name = 'Magnitude Out of Lim'
      | sbobj.Groups(4).Signals(7).XData = [0 0.724 0.991 1]
      | sbobj.Groups(4).Signals(7).YData = [0 0 0 0]
      | sbobj.Groups(4).Signals(8).Name = 'XY Out of Lim'
      | sbobj.Groups(4).Signals(8).XData = [0 0.777 0.992 1]
      | sbobj.Groups(4).Signals(8).YData = [0 0 0 0]
      | sbobj.Groups(4).Signals(9).Name = 'Overflow'
      | sbobj.Groups(4).Signals(9).XData = [0 0.831 0.992 1]
      | sbobj.Groups(4).Signals(9).YData = [0 0 0 0]
      | sbobj.Groups(4).Signals(10).Name = 'Voltage Fault'
      | sbobj.Groups(4).Signals(10).XData = [0 0.883 0.992 1]
      | sbobj.Groups(4).Signals(10).YData = [0 0 0 0]
      | sbobj.Groups(4).Signals(11).Name = 'IIF vs SSC Flt'
      | sbobj.Groups(4).Signals(11).XData = [0 0.4 0.6 1]
      | sbobj.Groups(4).Signals(11).YData = [0 0 0 0]
      | sbobj.Groups(4).Signals(12).Name = 'IIFvsSSC Offset'
      | sbobj.Groups(4).Signals(12).XData = [0 1]
      | sbobj.Groups(4).Signals(12).YData = [0 0]
      | sbobj.Groups(4).Signals(13).Name = 'TSFBit'
      | sbobj.Groups(4).Signals(13).XData = [0 0.4 0.6 1]
      | sbobj.Groups(4).Signals(13).YData = [0 0 0 0]
      | sbobj.Groups(4).Signals(14).Name = 'MotCtrlMotAgMecl0Polarity'
      | sbobj.Groups(4).Signals(14).XData = [0 1]
      | sbobj.Groups(4).Signals(14).YData = [-1 -1]
      | sbobj.Groups(4).TimeRange = [0 1]
      | sbobj.Groups(5).Name = 'Fault1'
      | sbobj.Groups(5).Signals(1).Name = 'Per1'
      | sbobj.Groups(5).Signals(1).XData = [0 0.026 0.026 0.028 1]
      | sbobj.Groups(5).Signals(1).YData = [0 0 1 1 1]
      | sbobj.Groups(5).Signals(2).Name = 'Per2'
      | sbobj.Groups(5).Signals(2).XData = [0 0.026 0.026 0.028 1]
      | sbobj.Groups(5).Signals(2).YData = [0 0 1 1 1]
      | sbobj.Groups(5).Signals(3).Name = 'Per3'
      | sbobj.Groups(5).Signals(3).XData = [0 0.026 0.026 0.05 1]
      | sbobj.Groups(5).Signals(3).YData = [0 0 1 1 1]
      | sbobj.Groups(5).Signals(4).Name = 'SPI Angle'
      | sbobj.Groups(5).Signals(4).XData = [0 1]
      | sbobj.Groups(5).Signals(4).YData = [1000 0]
      | sbobj.Groups(5).Signals(5).Name = 'No GMR Fault'
      | sbobj.Groups(5).Signals(5).XData = [0 0.122 0.122 0.15 0.15 1]
      | sbobj.Groups(5).Signals(5).YData = [0 0 1 1 0 0]
      | sbobj.Groups(5).Signals(6).Name = 'No Valid XY'
      | sbobj.Groups(5).Signals(6).XData = [0 0.259 0.259 0.272 0.272 1]
      | sbobj.Groups(5).Signals(6).YData = [0 0 1 1 0 0]
      | sbobj.Groups(5).Signals(7).Name = 'Magnitude Out of Lim'
      | sbobj.Groups(5).Signals(7).XData = [0 0.335 0.335 0.345 0.345 1]
      | sbobj.Groups(5).Signals(7).YData = [0 0 1 1 0 0]
      | sbobj.Groups(5).Signals(8).Name = 'XY Out of Lim'
      | sbobj.Groups(5).Signals(8).XData = [0 0.381 0.381 0.4 0.4 1]
      | sbobj.Groups(5).Signals(8).YData = [0 0 1 1 0 0]
      | sbobj.Groups(5).Signals(9).Name = 'Overflow'
      | sbobj.Groups(5).Signals(9).XData = [0 0.43 0.43 0.444 0.444 1]
      | sbobj.Groups(5).Signals(9).YData = [0 0 1 1 0 0]
      | sbobj.Groups(5).Signals(10).Name = 'Voltage Fault'
      | sbobj.Groups(5).Signals(10).XData = [0 0.473 0.473 0.49 0.49 1]
      | sbobj.Groups(5).Signals(10).YData = [0 0 1 1 0 0]
      | sbobj.Groups(5).Signals(11).Name = 'IIF vs SSC Flt'
      | sbobj.Groups(5).Signals(11).XData = [0 0.151 0.256 1]
      | sbobj.Groups(5).Signals(11).YData = [0 0 0 0]
      | sbobj.Groups(5).Signals(12).Name = 'IIFvsSSC Offset'
      | sbobj.Groups(5).Signals(12).XData = [0 1]
      | sbobj.Groups(5).Signals(12).YData = [2000 2000]
      | sbobj.Groups(5).Signals(13).Name = 'TSFBit'
      | sbobj.Groups(5).Signals(13).XData = [0 0.4 0.6 1]
      | sbobj.Groups(5).Signals(13).YData = [0 0 0 0]
      | sbobj.Groups(5).Signals(14).Name = 'MotCtrlMotAgMecl0Polarity'
      | sbobj.Groups(5).Signals(14).XData = [0 0.318 0.528 1]
      | sbobj.Groups(5).Signals(14).YData = [1 1 1 1]
      | sbobj.Groups(5).TimeRange = [0 1]
      | sbobj.Groups(6).Name = 'Offset Compensation'
      | sbobj.Groups(6).Signals(1).Name = 'Per1'
      | sbobj.Groups(6).Signals(1).XData = [0 0.028 1]
      | sbobj.Groups(6).Signals(1).YData = [1 1 1]
      | sbobj.Groups(6).Signals(2).Name = 'Per2'
      | sbobj.Groups(6).Signals(2).XData = [0 0.028 1]
      | sbobj.Groups(6).Signals(2).YData = [1 1 1]
      | sbobj.Groups(6).Signals(3).Name = 'Per3'
      | sbobj.Groups(6).Signals(3).XData = [0 0.028 1]
      | sbobj.Groups(6).Signals(3).YData = [1 1 1]
      | sbobj.Groups(6).Signals(4).Name = 'SPI Angle'
      | sbobj.Groups(6).Signals(4).XData = [0 1]
      | sbobj.Groups(6).Signals(4).YData = [0 1000]
      | sbobj.Groups(6).Signals(5).Name = 'No GMR Fault'
      | sbobj.Groups(6).Signals(5).XData = [0 0.122 0.122 0.15 0.15 1]
      | sbobj.Groups(6).Signals(5).YData = [0 0 1 1 0 0]
      | sbobj.Groups(6).Signals(6).Name = 'No Valid XY'
      | sbobj.Groups(6).Signals(6).XData = [0 0.259 0.259 0.272 0.272 1]
      | sbobj.Groups(6).Signals(6).YData = [0 0 1 1 0 0]
      | sbobj.Groups(6).Signals(7).Name = 'Magnitude Out of Lim'
      | sbobj.Groups(6).Signals(7).XData = [0 0.335 0.335 0.345 0.345 1]
      | sbobj.Groups(6).Signals(7).YData = [0 0 1 1 0 0]
      | sbobj.Groups(6).Signals(8).Name = 'XY Out of Lim'
      | sbobj.Groups(6).Signals(8).XData = [0 0.381 0.381 0.4 0.4 1]
      | sbobj.Groups(6).Signals(8).YData = [0 0 1 1 0 0]
      | sbobj.Groups(6).Signals(9).Name = 'Overflow'
      | sbobj.Groups(6).Signals(9).XData = [0 0.43 0.43 0.444 0.444 1]
      | sbobj.Groups(6).Signals(9).YData = [0 0 1 1 0 0]
      | sbobj.Groups(6).Signals(10).Name = 'Voltage Fault'
      | sbobj.Groups(6).Signals(10).XData = [0 0.473 0.473 0.49 0.49 1]
      | sbobj.Groups(6).Signals(10).YData = [0 0 1 1 0 0]
      | sbobj.Groups(6).Signals(11).Name = 'IIF vs SSC Flt'
      | sbobj.Groups(6).Signals(11).XData = [0 0.151 0.256 1]
      | sbobj.Groups(6).Signals(11).YData = [0 0 0 0]
      | sbobj.Groups(6).Signals(12).Name = 'IIFvsSSC Offset'
      | sbobj.Groups(6).Signals(12).XData = [0 1]
      | sbobj.Groups(6).Signals(12).YData = [98092.2 98092.2]
      | sbobj.Groups(6).Signals(13).Name = 'TSFBit'
      | sbobj.Groups(6).Signals(13).XData = [0 0.4 0.6 1]
      | sbobj.Groups(6).Signals(13).YData = [0 0 0 0]
      | sbobj.Groups(6).Signals(14).Name = 'MotCtrlMotAgMecl0Polarity'
      | sbobj.Groups(6).Signals(14).XData = [0 0.318 0.528 1]
      | sbobj.Groups(6).Signals(14).YData = [1 1 1 1]
      | sbobj.Groups(6).TimeRange = [0 1]
  Per1 : Outport  Tag=STV Outport
  Per2 : Outport  Tag=STV Outport  Port=2
  Per3 : Outport  Tag=STV Outport  Port=3
  SPI Angle : Outport  Tag=STV Outport  Port=4
  No GMR Fault : Outport  Tag=STV Outport  Port=5
  No Valid XY : Outport  Tag=STV Outport  Port=6
  Magnitude Out of Lim : Outport  Tag=STV Outport  Port=7
  XY Out of Lim : Outport  Tag=STV Outport  Port=8
  Overflow : Outport  Tag=STV Outport  Port=9
  Voltage Fault : Outport  Tag=STV Outport  Port=10
  IIF vs SSC Flt : Outport  Tag=STV Outport  Port=11
  IIFvsSSC Offset : Outport  Tag=STV Outport  Port=12
  TSFBit : Outport  Tag=STV Outport  Port=13
  MotCtrlMotAgMecl1Polarity : Outport  Tag=STV Outport  Port=14
  wires:
  FromWs/1 -> Demux/1
  Demux/1 -> Per1/1
  Demux/2 -> Per2/1
  Demux/3 -> Per3/1
  Demux/4 -> SPI Angle/1
  Demux/5 -> No GMR Fault/1
  Demux/6 -> No Valid XY/1
  Demux/7 -> Magnitude Out of Lim/1
  Demux/8 -> XY Out of Lim/1
  Demux/9 -> Overflow/1
  Demux/10 -> Voltage Fault/1
  Demux/11 -> IIF vs SSC Flt/1
  Demux/12 -> IIFvsSSC Offset/1
  Demux/13 -> TSFBit/1
  Demux/14 -> MotCtrlMotAgMecl1Polarity/1

== system CM640C_MotAg1Meas/MotAg1Meas/CopyRight2 ==

== system CM640C_MotAg1Meas/MotAg1Meas/MotAg1CoeffTblRead ==
  Trigger : TriggerPort  TriggerType=function-call  PortDimensions=1
  Copyright1 : Subsystem  Description=|  mask(Copyright Information){none=on}
      | Copyright info block.                                               
      |                                                                     
      | Place copyright information at the top of every subsystem in design.
      mask prompts: none "No parameters"
      mask help: Place copyright information at the top of every subsystem in design.
      mask Display:
      | NxtrConf = 'Nexteer Confidential';
      | 
      | sys = bdroot; %handle for the current model ("system")
      | first = get_param(sys,'Created');
      | if(isempty(first))
      |     first = datestr(now,'yyyy');
      | else
      |     first = first(end-3:end);  %year is last four digits
      | end
      | 
      | last = get_param(sys,'LastModifiedDate');
      | if isempty(last)
      |     last = datestr(now,'yyyy');
      | else
      |     last = last(end-3:end);
      | end
      | 
      | if strcmp(first,last)
      |     fprintf('%s\nCopyright  %s Nexteer',NxtrConf,first);
      | else
      |     fprintf('%s\n%s%s-%s Nexteer',NxtrConf,char(169),first,last);
      | end
  Data Store Read : DataStoreRead  DataStoreName=MotAg1CoeffTbl
  MotAgCoeffTbl_ArgOut : Outport
  wires:
  Data Store Read/1 -> MotAgCoeffTbl_ArgOut/1

== system CM640C_MotAg1Meas/MotAg1Meas/MotAg1CoeffTblWr ==
  MotAgCoeffTbl_ArgIn : Inport
  Trigger : TriggerPort  TriggerType=function-call  PortDimensions=1
  Block Changed = True : Constant  OutDataTypeStr=boolean
  Copyright1 : Subsystem  Description=|  mask(Copyright Information){none=on}
      | Copyright info block.                                               
      |                                                                     
      | Place copyright information at the top of every subsystem in design.
      mask prompts: none "No parameters"
      mask help: Place copyright information at the top of every subsystem in design.
      mask Display:
      | NxtrConf = 'Nexteer Confidential';
      | 
      | sys = bdroot; %handle for the current model ("system")
      | first = get_param(sys,'Created');
      | if(isempty(first))
      |     first = datestr(now,'yyyy');
      | else
      |     first = first(end-3:end);  %year is last four digits
      | end
      | 
      | last = get_param(sys,'LastModifiedDate');
      | if isempty(last)
      |     last = datestr(now,'yyyy');
      | else
      |     last = last(end-3:end);
      | end
      | 
      | if strcmp(first,last)
      |     fprintf('%s\nCopyright  %s Nexteer',NxtrConf,first);
      | else
      |     fprintf('%s\n%s%s-%s Nexteer',NxtrConf,char(169),first,last);
      | end
  Data Store Write : DataStoreWrite  DataStoreName=MotAg1CoeffTbl
  MotAg1CoeffTbl_SetRamBlockStatus : Subsystem
  wires:
  Block Changed = True/1 -> MotAg1CoeffTbl_SetRamBlockStatus/1(BlockChanged)
  MotAgCoeffTbl_ArgIn/1 -> Data Store Write/1

== system CM640C_MotAg1Meas/MotAg1Meas/MotAg1MeasInit1 ==
  function : TriggerPort  TriggerType=function-call
  Compute Correction Table : Subsystem  Priority=20  TreatAsAtomicUnit=on
      settings: AttributesFormatString=Priority = %<Priority>
  CopyRight2 : Subsystem  Description=|  mask(Copyright Information){none=on}
      | Copyright info block.                                               
      |                                                                     
      | Place copyright information at the top of every subsystem in design.
      mask prompts: none "No parameters"
      mask help: Place copyright information at the top of every subsystem in design.
      mask Display:
      | NxtrConf = 'Nexteer Confidential';
      | 
      | sys = bdroot; %handle for the current model ("system")
      | first = get_param(sys,'Created');
      | first = first(end-3:end);  %year is last four digits
      | 
      | last = get_param(sys,'LastModifiedDate');
      | if isempty(last)
      |     last = datestr(now,'yyyy');
      | else
      |     last = last(end-3:end);
      | end
      | 
      | if strcmp(first,last)
      |     fprintf('%s -- Copyright %s Nexteer',NxtrConf,first)
      | else
      |     fprintf('%s -- %s%s- %s Nexteer',NxtrConf,char(169),first,last)
      | end
  Initialize CSIH Registers and Start Transmission : Subsystem  RequirementInfo="{'linktype_rmi_doors' '00011b54 (/ESG Group/FDD Module Requirements/EA4 Specific/CM640C_MotAg1Meas)' '#CM640C_104' 'true' 'REQ:  CM640C_104' '' ; 'linktype_rmi_doors' '00011b54 (/ESG Group/FDD Module Requirements/EA4 Specific/CM640C_MotAg1Meas)' '#CM640C_111' 'true' 'REQ:  CM640C_111' '' } %GIDa_a35e1476_e7bc_4db2_abb6_e29bb2865be4"  Priority=10  TreatAsAtomicUnit=on
      settings: AttributesFormatString=Priority = %<Priority>

== system CM640C_MotAg1Meas/MotAg1Meas/MotAg1MeasPer1 ==
  MotCtrlMotAg1RtOffs : Inport  RequirementInfo={} %GIDa_a5b8bd2f_9c12_48b6_92fc_88f651d9a1ad
  function : TriggerPort  TriggerType=function-call
  CopyRight2 : Subsystem  Description=|  mask(Copyright Information){none=on}
      | Copyright info block.                                               
      |                                                                     
      | Place copyright information at the top of every subsystem in design.
      mask prompts: none "No parameters"
      mask help: Place copyright information at the top of every subsystem in design.
      mask Display:
      | NxtrConf = 'Nexteer Confidential';
      | 
      | sys = bdroot; %handle for the current model ("system")
      | first = get_param(sys,'Created');
      | first = first(end-3:end);  %year is last four digits
      | 
      | last = get_param(sys,'LastModifiedDate');
      | if isempty(last)
      |     last = datestr(now,'yyyy');
      | else
      |     last = last(end-3:end);
      | end
      | 
      | if strcmp(first,last)
      |     fprintf('%s -- Copyright %s Nexteer',NxtrConf,first)
      | else
      |     fprintf('%s -- %s%s- %s Nexteer',NxtrConf,char(169),first,last)
      | end
  Data Store Write : DataStoreWrite  DataStoreName=MotAg1Diagc
  Motor Angle Processing : Subsystem  RequirementInfo="{'linktype_rmi_doors' '00011b54 (/ESG Group/FDD Module Requirements/EA4 Specific/CM640C_MotAg1Meas)' '#CM640C_15' 'true' 'REQ:  CM640C_15' '' } %GIDa_ae90584e_6ea5_4d1a_8f19_fc25d0d64f41"
  MotCtrlMotAg1Mecl : Outport  RequirementInfo="{'linktype_rmi_doors' '00011b54 (/ESG Group/FDD Module Requirements/EA4 Specific/CM640C_MotAg1Meas)' '#CM640C_15' 'true' 'REQ:  CM640C_15' '' } %GIDa_7c3fa88b_712d_457b_9c0c_637aca600794"
  wires:
  Motor Angle Processing/1(MotCtrlMotAg1Mecl) -> Data Store Write/1, MotCtrlMotAg1Mecl/1
  MotCtrlMotAg1RtOffs/1 -> Motor Angle Processing/1(MotCtrlMotAg1Offs)

== system CM640C_MotAg1Meas/MotAg1Meas/MotAg1MeasPer2 ==
  MotAgMecl1Polarity : Inport
  MotAg4Mecl : Inport  Port=2
  MotAg1DiagcAg : Inport  Port=3
  MotAg1SpiTrsmEna : Inport  RequirementInfo={} %GIDa_9714a0c5_d169_4c20_b79a_08a62cfe6aba  Port=4
  function : TriggerPort  TriggerType=function-call
  CopyRight2 : Subsystem  Description=|  mask(Copyright Information){none=on}
      | Copyright info block.                                               
      |                                                                     
      | Place copyright information at the top of every subsystem in design.
      mask prompts: none "No parameters"
      mask help: Place copyright information at the top of every subsystem in design.
      mask Display:
      | NxtrConf = 'Nexteer Confidential';
      | 
      | sys = bdroot; %handle for the current model ("system")
      | first = get_param(sys,'Created');
      | first = first(end-3:end);  %year is last four digits
      | 
      | last = get_param(sys,'LastModifiedDate');
      | if isempty(last)
      |     last = datestr(now,'yyyy');
      | else
      |     last = last(end-3:end);
      | end
      | 
      | if strcmp(first,last)
      |     fprintf('%s -- Copyright %s Nexteer',NxtrConf,first)
      | else
      |     fprintf('%s -- %s%s- %s Nexteer',NxtrConf,char(169),first,last)
      | end
  MotAg1Calcn : Subsystem
  MotAg1MeclQlfr : Outport  RequirementInfo={} %GIDa_565f93ed_943b_4312_a87f_51762b2a2119
  MotAg1MeclRollgCntr : Outport  RequirementInfo={} %GIDa_8e528acc_6bf2_45f3_8e8a_135e746b0f24  Port=2
  MotAg1Offs : Outport  Port=3
  wires:
  MotAgMecl1Polarity/1 -> MotAg1Calcn/1(MotAgMecl1Polarity)
  MotAg4Mecl/1 -> MotAg1Calcn/2(MotAg4Mecl)
  MotAg1Calcn/1(MotAg1MeclQlfr) -> MotAg1MeclQlfr/1
  MotAg1Calcn/2(MotAg1MeclRollgCntr) -> MotAg1MeclRollgCntr/1
  MotAg1Calcn/3(MotAg1Offs) -> MotAg1Offs/1
  MotAg1SpiTrsmEna/1 -> MotAg1Calcn/Enable
  MotAg1DiagcAg/1 -> MotAg1Calcn/3(MotAg1DiagcAg)

== system CM640C_MotAg1Meas/MotAg1Meas/MotAg1MeasPer3 ==
  RegInpCSIH3STR0 : Inport
  function : TriggerPort  TriggerType=function-call
  CopyRight2 : Subsystem  Description=|  mask(Copyright Information){none=on}
      | Copyright info block.                                               
      |                                                                     
      | Place copyright information at the top of every subsystem in design.
      mask prompts: none "No parameters"
      mask help: Place copyright information at the top of every subsystem in design.
      mask Display:
      | NxtrConf = 'Nexteer Confidential';
      | 
      | sys = bdroot; %handle for the current model ("system")
      | first = get_param(sys,'Created');
      | first = first(end-3:end);  %year is last four digits
      | 
      | last = get_param(sys,'LastModifiedDate');
      | if isempty(last)
      |     last = datestr(now,'yyyy');
      | else
      |     last = last(end-3:end);
      | end
      | 
      | if strcmp(first,last)
      |     fprintf('%s -- Copyright %s Nexteer',NxtrConf,first)
      | else
      |     fprintf('%s -- %s%s- %s Nexteer',NxtrConf,char(169),first,last)
      | end
  Initial Check : Subsystem  RequirementInfo="{'linktype_rmi_doors' '00011b54 (/ESG Group/FDD Module Requirements/EA4 Specific/CM640C_MotAg1Meas)' '#CM640C_93' 'true' 'REQ:  CM640C_93' '' } %GIDa_f8bc9b8f_4d8d_43f3_8646_6df20ca79846"
  MotAg4Mecl : Outport
  MotAg1DiagcAg : Outport  Port=2
  MotAg1SpiTrsmEna : Outport  Port=3
  wires:
  RegInpCSIH3STR0/1 -> Initial Check/1(RegInpCSIH3STR0)
  Initial Check/1(MotAg4Mecl) -> MotAg4Mecl/1
  Initial Check/3(MotAg1SpiTrsmEna) -> MotAg1SpiTrsmEna/1
  Initial Check/2(MotAg1DiagcAg) -> MotAg1DiagcAg/1

== system CM640C_MotAg1Meas/Sensor Simulated Values/CopyRight2 ==

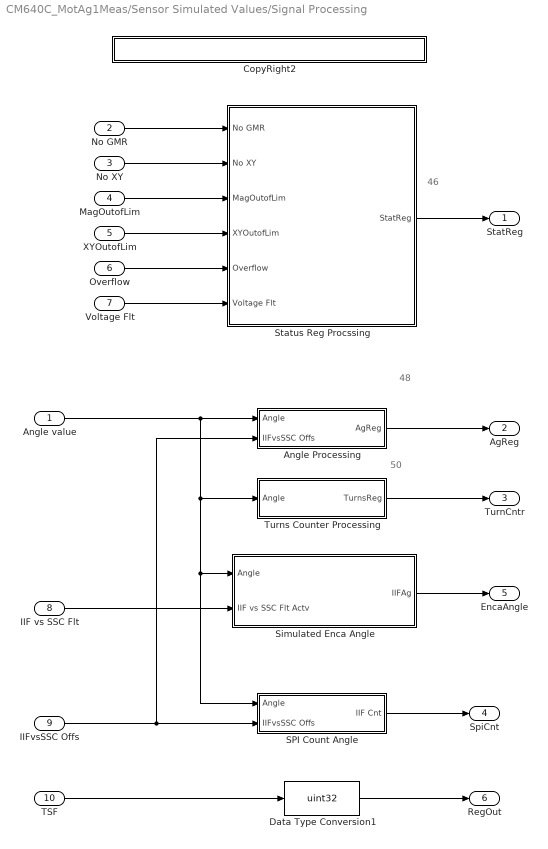
== system CM640C_MotAg1Meas/Sensor Simulated Values/Signal Processing ==
  note: 50
  note: 48
  note: 46
  Angle value : Inport
  No GMR : Inport  Port=2
  No XY : Inport  Port=3
  MagOutofLim : Inport  Port=4
  XYOutofLim : Inport  Port=5
  Overflow : Inport  Port=6
  Voltage Flt : Inport  Port=7
  IIF vs SSC Flt : Inport  Port=8
  IIFvsSSC Offs : Inport  Port=9
  TSF : Inport  Port=10
  Angle Processing : Subsystem
  CopyRight2 : Subsystem  Description=|  mask(Copyright Information){none=on}
      | Copyright info block.                                               
      |                                                                     
      | Place copyright information at the top of every subsystem in design.
      mask prompts: none "No parameters"
      mask help: Place copyright information at the top of every subsystem in design.
      mask Display:
      | NxtrConf = 'Nexteer Confidential';
      | 
      | sys = bdroot; %handle for the current model ("system")
      | first = get_param(sys,'Created');
      | first = first(end-3:end);  %year is last four digits
      | 
      | last = get_param(sys,'LastModifiedDate');
      | if isempty(last)
      |     last = datestr(now,'yyyy');
      | else
      |     last = last(end-3:end);
      | end
      | 
      | if strcmp(first,last)
      |     fprintf('%s -- Copyright %s Nexteer',NxtrConf,first)
      | else
      |     fprintf('%s -- %s%s- %s Nexteer',NxtrConf,char(169),first,last)
      | end
  Data Type Conversion1 : DataTypeConversion  OutDataTypeStr=uint32
  SPI Count Angle : Subsystem
  Simulated Enca Angle : Subsystem
  Status Reg Procssing : Subsystem
  Turns Counter Processing : Subsystem
  StatReg : Outport
  AgReg : Outport  Port=2
  TurnCntr : Outport  Port=3
  SpiCnt : Outport  Port=4
  EncaAngle : Outport  Port=5
  RegOut : Outport  Port=6
  wires:
  SPI Count Angle/1(IIF Cnt) -> SpiCnt/1
  Data Type Conversion1/1 -> RegOut/1
  Angle Processing/1(AgReg) -> AgReg/1
  IIFvsSSC Offs/1 -> Angle Processing/2(IIFvsSSC Offs), SPI Count Angle/2(IIFvsSSC Offs)
  Status Reg Procssing/1(StatReg) -> StatReg/1
  Turns Counter Processing/1(TurnsReg) -> TurnCntr/1
  TSF/1 -> Data Type Conversion1/1
  Overflow/1 -> Status Reg Procssing/5(Overflow)
  Voltage Flt/1 -> Status Reg Procssing/6(Voltage Flt)
  No GMR/1 -> Status Reg Procssing/1(No GMR)
  XYOutofLim/1 -> Status Reg Procssing/4(XYOutofLim)
  MagOutofLim/1 -> Status Reg Procssing/3(MagOutofLim)
  IIF vs SSC Flt/1 -> Simulated Enca Angle/2(IIF vs SSC Flt Actv)
  Simulated Enca Angle/1(IIFAg) -> EncaAngle/1
  No XY/1 -> Status Reg Procssing/2(No XY)
  Angle value/1 -> Simulated Enca Angle/1(Angle), SPI Count Angle/1(Angle), Turns Counter Processing/1(Angle), Angle Processing/1(Angle)

== system CM640C_MotAg1Meas/MotAg1Meas/MotAg1CoeffTblRead/Copyright1 ==

== system CM640C_MotAg1Meas/MotAg1Meas/MotAg1CoeffTblWr/Copyright1 ==

== system CM640C_MotAg1Meas/MotAg1Meas/MotAg1CoeffTblWr/MotAg1CoeffTbl_SetRamBlockStatus ==
  note: This is the block representing the client call
  BlockChanged : Inport
  Copyright1 : Subsystem  Description=|  mask(Copyright Information){none=on}
      | Copyright info block.                                               
      |                                                                     
      | Place copyright information at the top of every subsystem in design.
      mask prompts: none "No parameters"
      mask help: Place copyright information at the top of every subsystem in design.
      mask Display:
      | NxtrConf = 'Nexteer Confidential';
      | 
      | sys = bdroot; %handle for the current model ("system")
      | first = get_param(sys,'Created');
      | if(isempty(first))
      |     first = datestr(now,'yyyy');
      | else
      |     first = first(end-3:end);  %year is last four digits
      | end
      | 
      | last = get_param(sys,'LastModifiedDate');
      | if isempty(last)
      |     last = datestr(now,'yyyy');
      | else
      |     last = last(end-3:end);
      | end
      | 
      | if strcmp(first,last)
      |     fprintf('%s\nCopyright  %s Nexteer',NxtrConf,first);
      | else
      |     fprintf('%s\n%s%s-%s Nexteer',NxtrConf,char(169),first,last);
      | end
  Terminator : Terminator
  wires:
  BlockChanged/1 -> Terminator/1

== system CM640C_MotAg1Meas/MotAg1Meas/MotAg1MeasInit1/Compute Correction Table ==
  CopyRight2 : Subsystem  Description=|  mask(Copyright Information){none=on}
      | Copyright info block.                                               
      |                                                                     
      | Place copyright information at the top of every subsystem in design.
      mask prompts: none "No parameters"
      mask help: Place copyright information at the top of every subsystem in design.
      mask Display:
      | NxtrConf = 'Nexteer Confidential';
      | 
      | sys = bdroot; %handle for the current model ("system")
      | first = get_param(sys,'Created');
      | first = first(end-3:end);  %year is last four digits
      | 
      | last = get_param(sys,'LastModifiedDate');
      | if isempty(last)
      |     last = datestr(now,'yyyy');
      | else
      |     last = last(end-3:end);
      | end
      | 
      | if strcmp(first,last)
      |     fprintf('%s -- Copyright %s Nexteer',NxtrConf,first)
      | else
      |     fprintf('%s -- %s%s- %s Nexteer',NxtrConf,char(169),first,last)
      | end
  If : If  IfExpression=u1 == 0
  MotAg1CoeffTbl_GetErrorStatus : Subsystem  TreatAsAtomicUnit=on
  NVM NOK : Subsystem  TreatAsAtomicUnit=on
  NVM Ok : Subsystem  TreatAsAtomicUnit=on
  wires:
  MotAg1CoeffTbl_GetErrorStatus/1(RequestResultPtr) -> If/1
  If/1 -> NVM Ok/Action
  If/2 -> NVM NOK/Action

== system CM640C_MotAg1Meas/MotAg1Meas/MotAg1MeasInit1/CopyRight2 ==

== system CM640C_MotAg1Meas/MotAg1Meas/MotAg1MeasInit1/Initialize CSIH Registers and Start Transmission ==
  note: 1.  Configure the CSIH3 registers according to CM640C_MotAg1Meas_RegisterConfiguration.xlsm
      |     Order by Row.
  note: Follow below steps in same order:
      |
      | 1. Initialize CSIH Registers according to CM640C_MotAg1Meas_RegisterConfiguration.xlsm, Order by Row
      | 2. Start SPI Transmission by the mentioned Start pointer and No. of messeges
  note: CSIH3SOP - 0:6 bits (Start Pointer)
      | 000000 = 0
      | CSIH3ND 16:23 bits (No. Of Data)
      | 00001000 = 8
      | CSIH3BTST - 31st bit (Issue Transfer)
      | 1
      | Dec = 2148007936
  note: Tx Buffer ( 0 - 7)
  note: Send Tx Data in the following order. Start Pointer - Number of messeges.
  CopyRight2 : Subsystem  Description=|  mask(Copyright Information){none=on}
      | Copyright info block.                                               
      |                                                                     
      | Place copyright information at the top of every subsystem in design.
      mask prompts: none "No parameters"
      mask help: Place copyright information at the top of every subsystem in design.
      mask Display:
      | NxtrConf = 'Nexteer Confidential';
      | 
      | sys = bdroot; %handle for the current model ("system")
      | first = get_param(sys,'Created');
      | first = first(end-3:end);  %year is last four digits
      | 
      | last = get_param(sys,'LastModifiedDate');
      | if isempty(last)
      |     last = datestr(now,'yyyy');
      | else
      |     last = last(end-3:end);
      | end
      | 
      | if strcmp(first,last)
      |     fprintf('%s -- Copyright %s Nexteer',NxtrConf,first)
      | else
      |     fprintf('%s -- %s%s- %s Nexteer',NxtrConf,char(169),first,last)
      | end
  RegOutpCSIH3MCTL2 : Terminator
  "Start Pointer and No. of Data 2148007936 " : Constant  Value=STRTPTRINITVAL_CNT_U32
  wires:
  "Start Pointer and No. of Data 2148007936 "/1 -> RegOutpCSIH3MCTL2/1

== system CM640C_MotAg1Meas/MotAg1Meas/MotAg1MeasPer1/CopyRight2 ==

== system CM640C_MotAg1Meas/MotAg1Meas/MotAg1MeasPer1/Motor Angle Processing ==
  note: ENCA Client Call
  MotCtrlMotAg1Offs : Inport  RequirementInfo={} %GIDa_bd850cf1_7aad_4f85_9ca0_6a2ea660765b
  CopyRight2 : Subsystem  Description=|  mask(Copyright Information){none=on}
      | Copyright info block.                                               
      |                                                                     
      | Place copyright information at the top of every subsystem in design.
      mask prompts: none "No parameters"
      mask help: Place copyright information at the top of every subsystem in design.
      mask Display:
      | NxtrConf = 'Nexteer Confidential';
      | 
      | sys = bdroot; %handle for the current model ("system")
      | first = get_param(sys,'Created');
      | first = first(end-3:end);  %year is last four digits
      | 
      | last = get_param(sys,'LastModifiedDate');
      | if isempty(last)
      |     last = datestr(now,'yyyy');
      | else
      |     last = last(end-3:end);
      | end
      | 
      | if strcmp(first,last)
      |     fprintf('%s -- Copyright %s Nexteer',NxtrConf,first)
      | else
      |     fprintf('%s -- %s%s- %s Nexteer',NxtrConf,char(169),first,last)
      | end
  Data Store Write : DataStoreWrite  DataStoreName=dMotAg1MeasMotCtrlMotAg4Mecl
  GetMotAg4Mecl : Subsystem  RequirementInfo={} %GIDa_c1b4f818_c035_4912_a401_701e1761f0e3
  "Offset " : Subsystem  RequirementInfo="{'linktype_rmi_doors' '00011b54 (/ESG Group/FDD Module Requirements/EA4 Specific/CM640C_MotAg1Meas)' '#CM640C_77' 'true' 'REQ:  CM640C_77' '' } %GIDa_85691ae8_481c_4e23_b45f_e5d78164a88c"
  MotCtrlMotAg1Mecl : Outport
  wires:
  GetMotAg4Mecl/1(MotAgMecl) -> Data Store Write/1, "Offset "/1(MotAg4Mecl)
  MotCtrlMotAg1Offs/1 -> "Offset "/2(MotCtrlMotAg1Offs)
  "Offset "/1(MotCtrlMotAg1Mecl) -> MotCtrlMotAg1Mecl/1

== system CM640C_MotAg1Meas/MotAg1Meas/MotAg1MeasPer2/CopyRight2 ==

== system CM640C_MotAg1Meas/MotAg1Meas/MotAg1MeasPer2/MotAg1Calcn ==
  MotAgMecl1Polarity : Inport
  MotAg4Mecl : Inport  Port=2
  MotAg1DiagcAg : Inport  Port=3
  Enable : EnablePort
  CopyRight2 : Subsystem  Description=|  mask(Copyright Information){none=on}
      | Copyright info block.                                               
      |                                                                     
      | Place copyright information at the top of every subsystem in design.
      mask prompts: none "No parameters"
      mask help: Place copyright information at the top of every subsystem in design.
      mask Display:
      | NxtrConf = 'Nexteer Confidential';
      | 
      | sys = bdroot; %handle for the current model ("system")
      | first = get_param(sys,'Created');
      | first = first(end-3:end);  %year is last four digits
      | 
      | last = get_param(sys,'LastModifiedDate');
      | if isempty(last)
      |     last = datestr(now,'yyyy');
      | else
      |     last = last(end-3:end);
      | end
      | 
      | if strcmp(first,last)
      |     fprintf('%s -- Copyright %s Nexteer',NxtrConf,first)
      | else
      |     fprintf('%s -- %s%s- %s Nexteer',NxtrConf,char(169),first,last)
      | end
  MotAg1Processing : Subsystem
  SpiRx : Subsystem  TreatAsAtomicUnit=on
  MotAg1MeclQlfr : Outport  RequirementInfo={} %GIDa_565f93ed_943b_4312_a87f_51762b2a2119
  MotAg1MeclRollgCntr : Outport  RequirementInfo={} %GIDa_8e528acc_6bf2_45f3_8e8a_135e746b0f24  Port=2
  MotAg1Offs : Outport  Port=3
  wires:
  MotAgMecl1Polarity/1 -> MotAg1Processing/2(MotAgMecl1Polarity)
  MotAg4Mecl/1 -> MotAg1Processing/3(MotAg4Mecl)
  MotAg1Processing/1(MotAg1MeclQlfr) -> MotAg1MeclQlfr/1
  MotAg1Processing/2(MotAg1MeclRollgCntr) -> MotAg1MeclRollgCntr/1
  SpiRx/1(MotAg1RawRegBuf) -> MotAg1Processing/1(MotAg1RawRes)
  MotAg1Processing/3(MotAg1Offs) -> MotAg1Offs/1
  MotAg1DiagcAg/1 -> MotAg1Processing/4(MotAg1DiagcAg)

== system CM640C_MotAg1Meas/MotAg1Meas/MotAg1MeasPer3/CopyRight2 ==
